simulink model "ANS_GFM_long_term"  (R2021b)
settings: Solver=FixedStepAuto  StartTime=0.0  StopTime=160  FixedStep=Ts  MaxStep=1e-5  RelTol=1e-3
values from neighbouring files (symbols this model uses):
  angle_load = angle(LF.bus(ind_l).Vbus)*180/pi    [init_ANS_GFM_long_term.m]    (also in init_ANS_GFM_short_term.m)
  angleV_LF = Vangle_init/180*pi    [init_ANS_GFM_long_term.m]    (also in init_ANS_GFM_short_term.m)
  awu = 1    [init_ANS_GFM_long_term.m]    (also in init_ANS_GFM_short_term.m)
  C_dc = 1/(Xcdc_pu_or*Zbase_dc_new*100*pi)    [init_ANS_GFM_long_term.m]    (also in init_ANS_GFM_short_term.m)
  C_f = 1/(Xcf_pu_or*Zbase_new*100*pi)    (= 0.013712)    [init_ANS_GFM_long_term.m]    (also in init_ANS_GFM_short_term.m = 0.0141333333333)
  control = 3    [init_ANS_GFM_long_term.m]    (also in init_ANS_GFM_short_term.m = 1)
  D_p = (1/(m_p*w_b))    (= 5209935.26289)    [init_ANS_GFM_long_term.m]    (also in init_ANS_GFM_short_term.m = 5370022.73304)
  Egrid_tmp = 1.054080675694902*400e3    (= 421632.270278)    [init_ANS_GFM_long_term.m]    (also in init_ANS_GFM_short_term.m)
  epsi = 1e-4    (= 0.0001)    [init_ANS_GFM_long_term.m]    (also in init_ANS_GFM_short_term.m)
  eta = m_p*V_m^2    [init_ANS_GFM_long_term.m]    (also in init_ANS_GFM_short_term.m)
  gamma = 2.3    [init_ANS_GFM_long_term.m]    (also in init_ANS_GFM_short_term.m)
  I0_init = [I0_init_a, I0_init_b, I0_init_c]    [init_ANS_GFM_long_term.m]    (also in init_ANS_GFM_short_term.m)
  I_bc = S_bc / (V_bc*sqrt(3))    [init_ANS_GFM_long_term.m]    (also in init_ANS_GFM_short_term.m)
  I_d_int_init = (U_d_int + I_q_int*L_f*w_b - V_d_int - I_d_int*R_f*0)    [init_ANS_GFM_long_term.m]    (also in init_ANS_GFM_short_term.m)
  I_init = [I_init_a, I_init_b, I_init_c]    [init_ANS_GFM_long_term.m]    (also in init_ANS_GFM_short_term.m)
  i_ll = -1.15*(S_bc/Vdc_n)-i_loss_dc    [init_ANS_GFM_long_term.m]    (also in init_ANS_GFM_short_term.m)
  I_max_sat_pu = 1.0 * I_bc *sqrt(2)    [init_ANS_GFM_long_term.m]    (also in init_ANS_GFM_short_term.m)
  I_q_int_init = (U_q_int - I_d_int*L_f*w_b - V_q_int - I_q_int*R_f*0)    [init_ANS_GFM_long_term.m]    (also in init_ANS_GFM_short_term.m)
  i_ul = 1.15*(S_bc/Vdc_n)+i_loss_dc    [init_ANS_GFM_long_term.m]    (also in init_ANS_GFM_short_term.m)
  idppu = 0.95    [init_ANS_GFM_long_term.m]    (also in init_ANS_GFM_short_term.m = 0.92)
  init_dP = -inv(A_pm)*B_pm*dP    [init_ANS_GFM_long_term.m]    (also in init_ANS_GFM_short_term.m)
  init_pm = -inv(A_pm)*B_pm*P_aft    [init_ANS_GFM_long_term.m]    (also in init_ANS_GFM_short_term.m)
  init_tau = -inv(A_tau)*B_tau*idc    [init_ANS_GFM_long_term.m]    (also in init_ANS_GFM_short_term.m)
  init_v1 = 1.0    (= 1)    [init_ANS_GFM_long_term.m]    (also in init_ANS_GFM_short_term.m)
  init_v2 = abs(LF.bus(ind_g).Vbus)/sqrt(2)    [init_ANS_GFM_long_term.m]    (also in init_ANS_GFM_short_term.m)
  init_v3 = abs(LF.bus(ind_sg).Vbus)/sqrt(2)    [init_ANS_GFM_long_term.m]    (also in init_ANS_GFM_short_term.m)
  init_vload = 1.0    (= 1)    [init_ANS_GFM_long_term.m]    (also in init_ANS_GFM_short_term.m)
  J = D_p*tau_f    (= 104198.705258)    [init_ANS_GFM_long_term.m]    (also in init_ANS_GFM_short_term.m = 107400.454661)
  k_dc = eta_1/(Vdc_n*m_p)    [init_ANS_GFM_long_term.m]    (also in init_ANS_GFM_short_term.m)
  K_p = (1/Vdc_n)    [init_ANS_GFM_long_term.m]    (also in init_ANS_GFM_short_term.m)
  K_r = 1/R_dc    [init_ANS_GFM_long_term.m]    (also in init_ANS_GFM_short_term.m)
  Kff_i = 1    [init_ANS_GFM_long_term.m]    (also in init_ANS_GFM_short_term.m)
  Kff_v = 1    [init_ANS_GFM_long_term.m]    (also in init_ANS_GFM_short_term.m)
  Ki_i = (1/n)*1.19    (= 0.0520711785298)    [init_ANS_GFM_long_term.m]    (also in init_ANS_GFM_short_term.m = 0.0505188679245)
  Ki_pll = 4255.3    [init_ANS_GFM_long_term.m]    (also in init_ANS_GFM_short_term.m)
  Ki_v = (n)*1.161022    (= 26.5332227733)    [init_ANS_GFM_long_term.m]    (also in init_ANS_GFM_short_term.m = 27.3485182222)
  ki_v_ac = 2*0.25    (= 0.5)    [init_ANS_GFM_long_term.m]    (also in init_ANS_GFM_short_term.m)
  Kp_i = 0.738891/n    (= 0.032331869895)    [init_ANS_GFM_long_term.m]    (also in init_ANS_GFM_short_term.m = 0.0313680141509)
  Kp_pll = 92    [init_ANS_GFM_long_term.m]    (also in init_ANS_GFM_short_term.m)
  Kp_v = 0.52*n    (= 11.8837333333)    [init_ANS_GFM_long_term.m]    (also in init_ANS_GFM_short_term.m = 12.2488888889)
  kp_v_ac = 0.001    [init_ANS_GFM_long_term.m]    (also in init_ANS_GFM_short_term.m)
  Kpl = 5.0    (= 5)    [init_ANS_GFM_long_term.m]    (also in init_ANS_GFM_short_term.m)
  L1 = cf/sqrt(1+RX^2)*(400e3)^2/Skss/(100*pi)    [init_ANS_GFM_long_term.m]    (also in init_ANS_GFM_short_term.m)
  L_f = Xlf_pu_or*Zbase_new/100/pi    (= 4.37572928821e-06)    [init_ANS_GFM_long_term.m]    (also in init_ANS_GFM_short_term.m = 4.24528301887e-06)
  Lf = 1e6/100/pi    (= 3183.09886184)    [init_ANS_GFM_long_term.m]    (also in init_ANS_GFM_short_term.m = 0.0636619772368)
  m_p = (2*pi*0.5)/(S_bc)    (= 6.10967066042e-10)    [init_ANS_GFM_long_term.m]    (also in init_ANS_GFM_short_term.m = 5.92753330866e-10)
  n = 1/Zb    (= 22.8533333333)    [init_ANS_GFM_long_term.m]    (also in init_ANS_GFM_short_term.m = 23.5555555556)
  P_LF_si = P_LF*S_b    [init_ANS_GFM_long_term.m]    (also in init_ANS_GFM_short_term.m)
  ps = 4440e6/S_bc    (= 0.863477246208)    [init_ANS_GFM_long_term.m]    (also in init_ANS_GFM_short_term.m = 0.837735849057)
  Q_LF_si = Q_LF*S_b    [init_ANS_GFM_long_term.m]    (also in init_ANS_GFM_short_term.m)
  qs = Q_LF*S_b/S_bc    [init_ANS_GFM_long_term.m]    (also in init_ANS_GFM_short_term.m)
  R1 = RX*cf/sqrt(1+RX^2)*(400e3)^2/Skss    [init_ANS_GFM_long_term.m]    (also in init_ANS_GFM_short_term.m)
  R_dc = Rdc_pu_or*Zbase_dc_new    [init_ANS_GFM_long_term.m]    (also in init_ANS_GFM_short_term.m)
  R_f = Rf_pu_or*Zbase_new    (= 2.18786464411e-05)    [init_ANS_GFM_long_term.m]    (also in init_ANS_GFM_short_term.m = 2.12264150943e-05)
  Rf = 1e6    (= 1000000)    [init_ANS_GFM_long_term.m]    (also in init_ANS_GFM_short_term.m = 20)
  S_bc = 5142e6    (= 5142000000)    [init_ANS_GFM_long_term.m]    (also in init_ANS_GFM_short_term.m = 5300000000)
  sat_select = 3    [init_ANS_GFM_long_term.m]    (also in init_ANS_GFM_short_term.m)
  SECM = 3    [init_ANS_GFM_long_term.m]    (also in init_ANS_GFM_short_term.m = 1)
  share_i_load = 1.0    (= 1)    [init_ANS_GFM_long_term.m]    (also in init_ANS_GFM_short_term.m)
  T_en = -0.5    [init_ANS_GFM_long_term.m]    (also in init_ANS_GFM_short_term.m)
  T_off = T_on + 0.1    (= 0.2)    [init_ANS_GFM_long_term.m]    (also in init_ANS_GFM_short_term.m)
  T_on = 0.1    [init_ANS_GFM_long_term.m]    (also in init_ANS_GFM_short_term.m)
  Ts = 2e-6    (= 2e-06)    [init_ANS_GFM_long_term.m]    (also in init_ANS_GFM_short_term.m = 1e-06)
  U_init = [Umag_init_a, Umag_init_b, Umag_init_c]    [init_ANS_GFM_long_term.m]    (also in init_ANS_GFM_short_term.m)
  Uangle_init = angle(V_LF_VSC)*180/pi    [init_ANS_GFM_long_term.m]    (also in init_ANS_GFM_short_term.m)
  Umag_init = abs(V_LF_VSC)*V_bc*sqrt(2/3)    [init_ANS_GFM_long_term.m]    (also in init_ANS_GFM_short_term.m)
  V1_rms = 15e3    (= 15000)    [init_ANS_GFM_long_term.m]    (also in init_ANS_GFM_short_term.m)
  V_d_int = abs(V_LF)*V_bc*sqrt(2/3)    [init_ANS_GFM_long_term.m]    (also in init_ANS_GFM_short_term.m)
  V_d_int_init = (I_d_int + V_q_int*C_f*w_b - I0_d_int)    [init_ANS_GFM_long_term.m]    (also in init_ANS_GFM_short_term.m)
  V_init = [V_init_a, V_init_b, V_init_c]    [init_ANS_GFM_long_term.m]    (also in init_ANS_GFM_short_term.m)
  V_m = sqrt(2/3)*V_bc    [init_ANS_GFM_long_term.m]    (also in init_ANS_GFM_short_term.m)
  V_q_int_init = (I_q_int - V_d_int*C_f*w_b - I0_q_int)    [init_ANS_GFM_long_term.m]    (also in init_ANS_GFM_short_term.m)
  Vdc_n = 3*V_m    [init_ANS_GFM_long_term.m]    (also in init_ANS_GFM_short_term.m)
  Vref = V_LF_mag*V_m    [init_ANS_GFM_long_term.m]    (also in init_ANS_GFM_short_term.m)
  w_b = 2*pi*f_b    (= 314.159265359)    [init_ANS_GFM_long_term.m]    (also in init_ANS_GFM_short_term.m)
  w_f = 2*pi*5    (= 31.4159265359)    [init_ANS_GFM_long_term.m]    (also in init_ANS_GFM_short_term.m)
  Zbase_new = V1_rms^2/S_bc    (= 0.0437572928821)    [init_ANS_GFM_long_term.m]    (also in init_ANS_GFM_short_term.m = 0.0424528301887)
undefined symbols (not defined in the file or in its folder): A_pm, A_tau, B_pm, B_tau, C_pm, C_tau, D_pm, D_tau, find_system, idq0_init, Pm, sm_init, v_d, v_q, Ve
libraries: spsBreakerLib x135, spsGroundLib x18, spsThreePhaseSeriesRLCBranchLib x12, spsabctodq0Lib x11, simulink x9, spsThreePhaseVIMeasurementLib x7, spsLoadFlowBusLib x7, spsSeriesRLCBranchLib x6, spsControlledVoltageSourceLib x6, spsCurrentMeasurementLib x6, spsVoltageMeasurementLib x6, spsRMSLib x5
(part 2 of 5)

== system ANS_GFM_long_term/OLTC ==
  note: G. Sybille, P. Giroux Hydro-Quebec (IREQ)
  note: This Three-Phase OLTC Regulating Transformer is built with three Multi-Winding Transformer blocks
      | and three On-Load Tap Changers (OLTC) subsystems using switches.
      | It implements a fixed number of taps (8 taps per phase +  tap 0 (nominal voltage ratio)).
      |
      | In order to change the number of taps you must modify the 3 Transformer blocks
      | and the 3  OLTC blocks as explained in the  the procedure given below:
  Vm (pu) : Inport
  " OLTC Control" : Subsystem  mask{NumberOfTaps=NumberOfTaps, TapSelectionTime=TapSelectionTime, TransferTime=TransferTime, InitialTap=InitialTap}
      mask prompts: NumberOfTaps "Number of taps:"; TapSelectionTime "Operating time of the tap selector (typical 3-10 s):"; TransferTime "Operating time of the transfer switch (typical 40-60 ms):"; InitialTap "Initial tap:"
      mask init:
      | TapVector=0:NumberOfTaps;
      | InitialStates=zeros(1,NumberOfTaps+1);
  Constant : Constant  Value=RegulatorOn
  Display : Display  Commented=on
  Goto Tag Visibility : GotoTagVisibility  GotoTag=SwSelect
  Goto Tag Visibility1 : GotoTagVisibility  GotoTag=SwTransfer
  Goto Tag Visibility2 : GotoTagVisibility  GotoTag=SwInversion
  Ground : spsGroundLib/Ground  LConnTagsString=a
  Ground1 : spsGroundLib/Ground  LConnTagsString=a
  Ground2 : spsGroundLib/Ground  LConnTagsString=a
  OLTCA : Subsystem  mask{NumberOfTaps=NumberOfTaps, InitialTap=InitialTap, Rtransfer=Rtransfer}
      mask prompts: NumberOfTaps "Nombre de prises:"; InitialTap "Prise initiale:"; Rtransfer "Resistance de court circuit (ohms):"
      mask init:
      | TapVector=0:NumberOfTaps;
      | InitialStates=zeros(1,NumberOfTaps+1);
      | InitialStates(abs(InitialTap)+1)=1;
      | 
      | InitialStateInv1=(InitialTap>=0);
      | InitialStateInv2=(InitialTap<0);
      | InitialStateInv3=InitialStateInv1;
      | InitialStateInv4=InitialStateInv2;
  OLTCA1 : Subsystem  mask{NumberOfTaps=NumberOfTaps, InitialTap=InitialTap, Rtransfer=Rtransfer}
      mask prompts: NumberOfTaps "Nombre de prises:"; InitialTap "Prise initiale:"; Rtransfer "Resistance de court circuit (ohms):"
      mask init: same as ANS_GFM_long_term/OLTC/OLTCA
  OLTCA2 : Subsystem  mask{NumberOfTaps=NumberOfTaps, InitialTap=InitialTap, Rtransfer=Rtransfer}
      mask prompts: NumberOfTaps "Nombre de prises:"; InitialTap "Prise initiale:"; Rtransfer "Resistance de court circuit (ohms):"
      mask init: same as ANS_GFM_long_term/OLTC/OLTCA
  OLTCA3 : Subsystem  Commented=on  mask{NumberOfTaps=NumberOfTaps, InitialTap=InitialTap, Rtransfer=Rtransfer}
      mask prompts: NumberOfTaps "Nombre de prises:"; InitialTap "Prise initiale:"; Rtransfer "Resistance de court circuit (ohms):"
      mask init: same as ANS_GFM_long_term/OLTC/OLTCA
  OLTCC1 : Subsystem  Commented=on  mask{NumberOfTaps=NumberOfTaps, InitialTap=InitialTap, Rtransfer=Rtransfer}
      mask prompts: NumberOfTaps "Nombre de prises:"; InitialTap "Prise initiale:"; Rtransfer "Resistance de court circuit (ohms):"
      mask init: same as ANS_GFM_long_term/OLTC/OLTCA
  Subsystem : Subsystem
      mask Display: disp('Procedure\n to change\n the number of taps')
  TransformerA : spsMultiWindingTransformerLib/Multi-Winding Transformer  LeftWindings=1  RightWindings=2  TappedWindings=taps on upper right winding  NumberOfTaps=19  SetSaturation=off  Hysteresis=off  DataFile='hysteresis.mat'  Measurements=None  UNITS=pu  NominalPower="[Pnom  Fnom]"  NominalVoltages=[Vnom1 VnomTaps Vnom2 ]  WindingResistances=[Rpu1 RpuTaps Rpu2]  WindingInductances="[Xpu1 XpuTaps  Xpu2 ]"  Rm=Rm  Lm=Lm  Saturation=[ 0,0 ; 0.0024,1.2 ; 1.0,1.52 ]  BreakLoop=off  DiscreteSolver=Trapezoidal iterative  DataType=off  InitialFlux=0  TransfoNumber=1
      settings: SourceProductBaseCode=PS
  TransformerB : spsMultiWindingTransformerLib/Multi-Winding Transformer  LeftWindings=1  RightWindings=2  TappedWindings=taps on upper right winding  NumberOfTaps=19  SetSaturation=off  Hysteresis=off  DataFile='hysteresis.mat'  Measurements=None  UNITS=pu  NominalPower="[Pnom  Fnom]"  NominalVoltages=[Vnom1 VnomTaps Vnom2 ]  WindingResistances=[Rpu1 RpuTaps Rpu2]  WindingInductances="[Xpu1 XpuTaps  Xpu2 ]"  Rm=Rm  Lm=Lm  Saturation=[ 0,0 ; 0.0024,1.2 ; 1.0,1.52 ]  BreakLoop=off  DiscreteSolver=Trapezoidal iterative  DataType=off  InitialFlux=0  TransfoNumber=1
      settings: SourceProductBaseCode=PS
  TransformerC : spsMultiWindingTransformerLib/Multi-Winding Transformer  LeftWindings=1  RightWindings=2  TappedWindings=taps on upper right winding  NumberOfTaps=19  SetSaturation=off  Hysteresis=off  DataFile='hysteresis.mat'  Measurements=None  UNITS=pu  NominalPower="[Pnom  Fnom]"  NominalVoltages=[Vnom1 VnomTaps Vnom2 ]  WindingResistances=[Rpu1 RpuTaps Rpu2]  WindingInductances="[Xpu1 XpuTaps  Xpu2 ]"  Rm=Rm  Lm=Lm  Saturation=[ 0,0 ; 0.0024,1.2 ; 1.0,1.52 ]  BreakLoop=off  DiscreteSolver=Trapezoidal iterative  DataType=off  InitialFlux=0  TransfoNumber=1
      settings: SourceProductBaseCode=PS
  Voltage regulator : Subsystem  mask{Vref=RegulatorVref, DeadBand=RegulatorDeadBand, TimeDelay=RegulatorDelay}
      mask prompts: Vref "Vref (pu)"; DeadBand "Deadband (pu)"; TimeDelay "Time delay (s)"
  A : PMIOPort  Tag=PMCPort  Side=Left
  B : PMIOPort  Tag=PMCPort  Port=2  Side=Left
  C : PMIOPort  Tag=PMCPort  Port=3  Side=Left
  a : PMIOPort  Tag=PMCPort  Port=4  Side=Right
  b : PMIOPort  Tag=PMCPort  Port=5  Side=Right
  c : PMIOPort  Tag=PMCPort  Port=6  Side=Right
  Tap : Outport  VectorParamsAs1DForOutWhenUnconnected=off
  tag scope: SwInversion=scoped, SwSelect=scoped, SwTransfer=scoped
  wires:
  Constant/1 -> Voltage regulator/3(RegOn)
  Vm (pu)/1 -> Voltage regulator/1(Vmes (pu))
  Voltage regulator/2(Down) -> " OLTC Control"/2(Down)
  " OLTC Control"/5(Ready) -> Voltage regulator/2(Ready)
  Voltage regulator/1(Up) -> " OLTC Control"/1(Up)
  " OLTC Control"/4(SwInv) -> [SwInversion]
  " OLTC Control"/1(Tap) -> Display/1, Tap/1  "Tap"
  " OLTC Control"/2(SwSelect) -> [SwSelect]
  " OLTC Control"/3(SwTr) -> [SwTransfer]
  connections:
  OLTCA/RConn22 -- TransformerA/RConn22
  OLTCA/RConn21 -- TransformerA/RConn21
  OLTCA/RConn20 -- TransformerA/RConn20
  OLTCA/RConn19 -- TransformerA/RConn19
  OLTCA/RConn18 -- TransformerA/RConn18
  OLTCA/RConn17 -- TransformerA/RConn17
  OLTCA/RConn16 -- TransformerA/RConn16
  OLTCA/RConn15 -- TransformerA/RConn15
  OLTCA/RConn13 -- TransformerA/RConn13
  OLTCA/RConn12 -- TransformerA/RConn12
  OLTCA/RConn14 -- TransformerA/RConn14
  OLTCA/RConn11 -- TransformerA/RConn11
  OLTCA/RConn10 -- TransformerA/RConn10
  OLTCA/RConn9 -- TransformerA/RConn9
  OLTCA/RConn8 -- TransformerA/RConn8
  OLTCA/RConn7 -- TransformerA/RConn7
  OLTCA/RConn6 -- TransformerA/RConn6
  OLTCA/RConn5 -- TransformerA/RConn5
  OLTCA/RConn4 -- TransformerA/RConn4
  OLTCA/RConn3 -- TransformerA/RConn3
  OLTCA/RConn2 -- TransformerA/RConn2
  OLTCA/RConn1 -- TransformerA/RConn1
  Ground/LConn1 -- TransformerA/RConn23
  OLTCA/LConn1 -- a/RConn1
  Ground1/LConn1 -- TransformerB/RConn23
  OLTCA1/RConn7 -- TransformerB/RConn7
  OLTCA1/RConn17 -- TransformerB/RConn17
  OLTCA1/RConn21 -- TransformerB/RConn21
  OLTCA1/RConn15 -- TransformerB/RConn15
  OLTCA1/RConn14 -- TransformerB/RConn14
  OLTCA1/RConn3 -- TransformerB/RConn3
  OLTCA1/RConn9 -- TransformerB/RConn9
  OLTCA1/RConn13 -- TransformerB/RConn13
  OLTCA1/RConn8 -- TransformerB/RConn8
  OLTCA1/RConn1 -- TransformerB/RConn1
  OLTCA1/RConn16 -- TransformerB/RConn16
  OLTCA1/RConn12 -- TransformerB/RConn12
  OLTCA1/RConn4 -- TransformerB/RConn4
  OLTCA1/RConn5 -- TransformerB/RConn5
  OLTCA1/RConn2 -- TransformerB/RConn2
  OLTCA1/RConn10 -- TransformerB/RConn10
  OLTCA1/RConn6 -- TransformerB/RConn6
  OLTCA1/RConn20 -- TransformerB/RConn20
  OLTCA1/RConn22 -- TransformerB/RConn22
  OLTCA1/RConn18 -- TransformerB/RConn18
  OLTCA1/RConn19 -- TransformerB/RConn19
  OLTCA1/RConn11 -- TransformerB/RConn11
  Ground2/LConn1 -- TransformerC/RConn23
  OLTCA2/RConn7 -- TransformerC/RConn7
  OLTCA2/RConn17 -- TransformerC/RConn17
  OLTCA2/RConn21 -- TransformerC/RConn21
  OLTCA2/RConn15 -- TransformerC/RConn15
  OLTCA2/RConn14 -- TransformerC/RConn14
  OLTCA2/RConn3 -- TransformerC/RConn3
  OLTCA2/RConn9 -- TransformerC/RConn9
  OLTCA2/RConn13 -- TransformerC/RConn13
  OLTCA2/RConn8 -- TransformerC/RConn8
  OLTCA2/RConn1 -- TransformerC/RConn1
  OLTCA2/RConn16 -- TransformerC/RConn16
  OLTCA2/RConn12 -- TransformerC/RConn12
  OLTCA2/RConn4 -- TransformerC/RConn4
  OLTCA2/RConn5 -- TransformerC/RConn5
  OLTCA2/RConn2 -- TransformerC/RConn2
  OLTCA2/RConn10 -- TransformerC/RConn10
  OLTCA2/RConn6 -- TransformerC/RConn6
  OLTCA2/RConn20 -- TransformerC/RConn20
  OLTCA2/RConn22 -- TransformerC/RConn22
  OLTCA2/RConn18 -- TransformerC/RConn18
  OLTCA2/RConn19 -- TransformerC/RConn19
  OLTCA2/RConn11 -- TransformerC/RConn11
  OLTCA2/LConn1 -- c/RConn1
  OLTCA1/LConn1 -- b/RConn1
  TransformerA/LConn2 -- TransformerB/LConn1 -- B/RConn1
  TransformerB/LConn2 -- C/RConn1 -- TransformerC/LConn1
  TransformerC/LConn2 -- A/RConn1 -- TransformerA/LConn1

== system ANS_GFM_long_term/Synchronous Generator(GENTPJ) ==
  ve : Inport
  Pm : Inport  Port=2
  AVR+OEL+PSS : Subsystem  mask(AVR){ve0=Ve, uref=1.0, ifdlim=3.0618, L1=-20, L2=5, G=120, Ta=5, Tb=12.5, PSS_act=1, Kp=75, Tw=15, T1=0.22, T2=0.012, C=0.1}
      mask prompts: ve0 "Initialisierung Erregerspannung (ve0)"; uref "Referenzklemmenspannung (uref)"; ifdlim "max. Erregerstrom (ifdlim)"; L1 "Over-Excitation Limit (L1)"; L2 "AVR Limit (L2)"; G "Verstärkungsfaktor (G)"; Ta "AVR Zeitkonstante (Ta)"; Tb "AVR Zeitkonstante (Tb)"; PSS_act "PSS on/off (1/0)"; Kp "Verstärkungsfaktor PSS"; Tw "Wash-Out Filter (Tw)"; T1 "PSS Zeitkonstante (T1)"; T2 "PSS Zeitkonstante (T2)"; C "PSS Begrenzung"
      mask help: AVR
  Grid Interface : Subsystem
  Mechanical Equations : Subsystem
  Power calculation : Subsystem
  Rotor Equations : Subsystem
  Stator Equations : Subsystem
  Terminator : Terminator
  To Workspace1 : ToWorkspace  VariableName=psm  SampleTime=-1
      settings: Decimation=100
  To Workspace2 : ToWorkspace  VariableName=ifdsm  SampleTime=-1
      settings: Decimation=100
  a : PMIOPort  Side=Right
  b : PMIOPort  Port=2  Side=Right
  c : PMIOPort  Port=3  Side=Right
  delta : Outport
  wt : Outport  Port=2
  wires:
  Mechanical Equations/1(1+w) -> AVR+OEL+PSS/3(xspeed), Stator Equations/6(1+w), Power calculation/1(1+w)
  Stator Equations/2(Vqterm) -> Grid Interface/2(Vqterm), Power calculation/3(Vqterm)
  Power calculation/1(Te) -> To Workspace1/1, Mechanical Equations/2(Te)
  Rotor Equations/1(ifd) -> AVR+OEL+PSS/1(ie), To Workspace2/1
  Mechanical Equations/2(wt) -> Grid Interface/3(wt), wt/1
  Mechanical Equations/3(delta) -> delta/1
  Pm/1 -> Mechanical Equations/1(Pm)
  Rotor Equations/2(Edss) -> Stator Equations/3(Edss)
  Rotor Equations/3(Eqss) -> Stator Equations/4(Eqss)
  Grid Interface/1(id) -> Power calculation/4(Id), Stator Equations/1(Id), Rotor Equations/2(id)
  Grid Interface/2(iq) -> Power calculation/5(Iq), Stator Equations/2(Iq), Rotor Equations/3(iq)
  Grid Interface/4(|Uterm|) -> AVR+OEL+PSS/2(ut)
  ve/1 -> Terminator/1
  Stator Equations/1(Vdterm) -> Grid Interface/1(Vdterm), Power calculation/2(Vdterm)  "Eqs"
  Grid Interface/3(El) -> Stator Equations/5(E_l), Rotor Equations/4(El)
  AVR+OEL+PSS/1(ve) -> Rotor Equations/1(ve)
  connections:
  Grid Interface/RConn1 -- a/RConn1
  Grid Interface/RConn3 -- c/RConn1
  Grid Interface/RConn2 -- b/RConn1

== system ANS_GFM_long_term/Constant Current Load (EMT)/PLL ==
  Vabc : Inport
  Constant1 : Constant  Value=sqrt(2)*Pload/(sqrt(3)*Urms)
  Constant2 : Constant  Value=0
  Constant4 : Constant  Value=100*pi
  Cos : Trigonometry  Operator=cos
  Cos1 : Trigonometry
  Demux1 : Demux  Outputs=3
  Demux2 : Demux  Outputs=3
  Gain4 : Gain  Gain=Ki
  Gain5 : Gain  Gain=Kp
  Integrator2 : Integrator  InitialCondition=angle_load/180*pi-pi/2
  Integrator3 : Integrator
  Mux : Mux  Inputs=3
  Product : Product
  Product1 : Product
  Saturation1 : Saturate  UpperLimit=2*pi*55  LowerLimit=2*pi*45
  Sum2 : Sum  Inputs=|++
  Sum3 : Sum  Inputs=|++
  Sum4 : Sum  Inputs=-+
  Terminator : Terminator
  abc to Alpha-Beta-Zero : spsabctoAlphaBetaZeroLib/abc to Alpha-Beta-Zero
      settings: SourceProductBaseCode=PS
  delay : TransferFcn  Denominator=[Ts 1]
  dq0 to abc : spsdq0toabcLib/dq0 to abc  Alignment=Aligned with phase A axis
  Ia : Outport
  Ib : Outport  Port=2
  Ic : Outport  Port=3
  wires:
  Demux1/1 -> Ia/1
  Demux1/2 -> Ib/1
  Mux/1 -> dq0 to abc/1
  dq0 to abc/1 -> Demux1/1
  Demux1/3 -> Ic/1
  Constant2/1 -> Mux/2, Mux/3
  Constant1/1 -> Mux/1
  abc to Alpha-Beta-Zero/1 -> Demux2/1
  Sum2/1 -> Sum3/1
  Integrator3/1 -> Sum2/2
  Saturation1/1 -> Integrator2/1
  Gain5/1 -> Sum2/1
  Sum3/1 -> Saturation1/1
  Gain4/1 -> Integrator3/1
  Constant4/1 -> Sum3/2
  Product/1 -> Sum4/1
  Product1/1 -> Sum4/2
  Integrator2/1 -> Cos1/1, Cos/1, dq0 to abc/2
  Cos/1 -> Product1/2
  Cos1/1 -> Product/1
  Vabc/1 -> abc to Alpha-Beta-Zero/1
  Demux2/1 -> Product/2
  Demux2/2 -> Product1/1
  Sum4/1 -> delay/1
  delay/1 -> Gain4/1, Gain5/1
  Demux2/3 -> Terminator/1

== system ANS_GFM_long_term/GFM Converter/Converter (modified by S. Liemann) ==
  note: AC sources
  Vdq0 : Inport
  Pe_ac : Inport  Port=2
  Idc : Inport  Port=3
  wt : Inport  Port=4
  Divide : Product  Inputs=*/
  Gain12 : Gain  Gain=1/C_dc
  Gain13 : Gain  Gain=1/R_dc
  Gain8 : Gain  Gain=1/Vdc_n
  Integrator1 : Integrator  InitialCondition=Vdc_n
  Product5 : Product
  Subsystem1 : Subsystem
  Sum3 : Sum  Inputs=-+-
  dq0 to abc1 : spsdq0toabcLib/dq0 to abc  Alignment=90 degrees behind phase A axis
  a : PMIOPort  Side=Right
  b : PMIOPort  Port=2  Side=Right
  c : PMIOPort  Port=3  Side=Right
  Udc : Outport
  wires:
  Integrator1/1 -> Gain8/1, Divide/2, Udc/1, Gain13/1  "Udc"
  wt/1 -> dq0 to abc1/2
  Product5/1 -> dq0 to abc1/1
  Sum3/1 -> Gain12/1  "Ic"
  dq0 to abc1/1 -> Subsystem1/1(Vabc)
  Idc/1 -> Sum3/2
  Gain12/1 -> Integrator1/1
  Gain13/1 -> Sum3/3
  Vdq0/1 -> Product5/1
  Pe_ac/1 -> Divide/1
  Divide/1 -> Sum3/1
  Gain8/1 -> Product5/2
  connections:
  Subsystem1/RConn2 -- b/RConn1
  Subsystem1/RConn1 -- a/RConn1
  Subsystem1/RConn3 -- c/RConn1

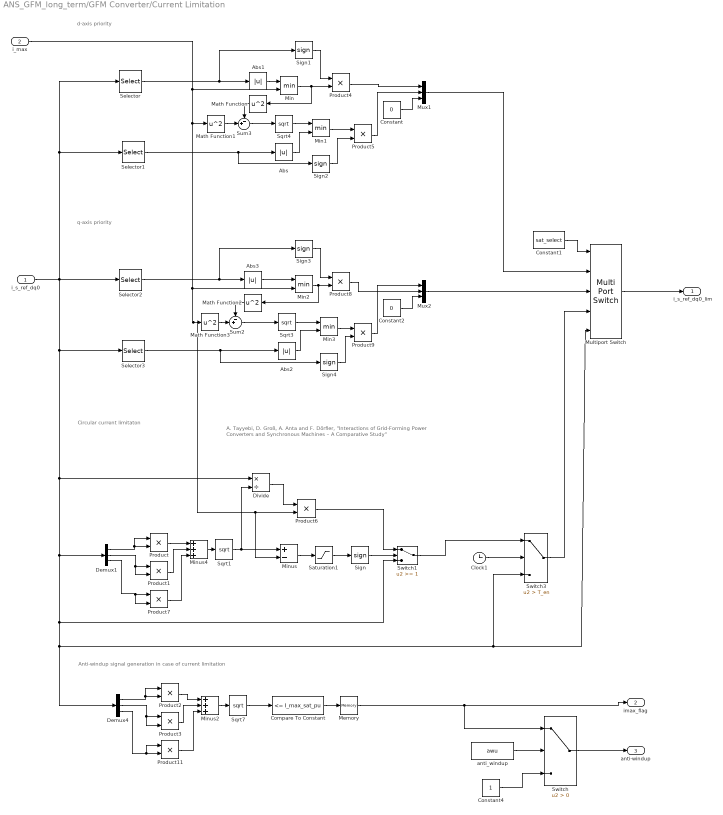
== system ANS_GFM_long_term/GFM Converter/Current Limitation ==
  note: Anti-windup signal generation in case of current limitation
  note: d-axis priority
  note: Circular current limitaton
  note: A. Tayyebi, D. Groß, A. Anta and F. Dörfler, "Interactions of Grid-Forming Power Converters and Synchronous Machines – A Comparative Study"
  note: q-axis priority
  i_s_ref_dq0 : Inport
  i_max : Inport  Port=2
  Abs{,1..3} (4 alike) : Abs
  Clock1 : Clock
  Compare To Constant : simulink/Logic and Bit Operations/Compare To Constant  relop=<=  const=I_max_sat_pu  OutDataTypeStr=boolean
  Constant : Constant  Value=0
  Constant1 : Constant  Value=sat_select
  Constant2 : Constant  Value=0
  Constant4 : Constant
  Demux1 : Demux  Outputs=3
  Demux4 : Demux  Outputs=3
  Divide : Product  Inputs=*/
  Math Function{,1..3} (4 alike) : Math  Operator=square  SaturateOnIntegerOverflow=on
  Memory : Memory  InitialCondition=1
  Min{,1..3} (4 alike) : MinMax  Inputs=2
  Minus : Sum  Inputs=+-
  Minus2 : Sum  Inputs=+++
  Minus4 : Sum  Inputs=+++
  Multiport Switch : MultiPortSwitch  Inputs=4
  Mux1 : Mux  Inputs=3
  Mux2 : Mux  Inputs=3
  Product{,1..3,6..7,11} (7 alike) : Product  RndMeth=Zero
  Product{4..5,8..9} (4 alike) : Product
  Saturation1 : Saturate  UpperLimit=inf  LowerLimit=0
  Selector : Selector  InputPortWidth=3  IndexOptions=Index vector (dialog)  Indices=[1 ]  OutputSizes=1
  Selector1 : Selector  InputPortWidth=3  IndexOptions=Index vector (dialog)  Indices=[2 ]  OutputSizes=1
  Selector2 : Selector  InputPortWidth=3  IndexOptions=Index vector (dialog)  Indices=[2 ]  OutputSizes=1
  Selector3 : Selector  InputPortWidth=3  IndexOptions=Index vector (dialog)  Indices=[1 ]  OutputSizes=1
  Sign{,1..4} (5 alike) : Signum
  Sqrt{1,3..4,7} (4 alike) : Sqrt  SaturateOnIntegerOverflow=on
  Sum2 : Sum  Inputs=-+|
  Sum3 : Sum  Inputs=-+|
  Switch : Switch  Criteria=u2 > Threshold
  Switch1 : Switch  Threshold=1
  Switch3 : Switch  Criteria=u2 > Threshold  Threshold=T_en
  anti_windup : Constant  Value=awu
  i_s_ref_dq0_lim : Outport  VectorParamsAs1DForOutWhenUnconnected=off
  imax_flag : Outport  Port=2
  anti-windup : Outport  Port=3
  wires:
  Demux1/3 -> Product7/2, Product7/1
  Product/1 -> Minus4/1
  Demux1/2 -> Product1/2, Product1/1
  Sqrt1/1 -> Minus/1, Divide/2
  Minus/1 -> Saturation1/1
  Demux1/1 -> Product/1, Product/2
  Product1/1 -> Minus4/2
  Minus4/1 -> Sqrt1/1
  Divide/1 -> Product6/1
  Saturation1/1 -> Sign/1
  Sign/1 -> Switch1/2
  Product7/1 -> Minus4/3
  Product6/1 -> Switch1/1
  Selector/1 -> Sign1/1, Abs1/1
  Sqrt4/1 -> Min1/1
  Sum3/1 -> Sqrt4/1
  Constant/1 -> Mux1/3
  Constant1/1 -> Multiport Switch/1
  Mux1/1 -> Multiport Switch/2
  Abs/1 -> Min1/2
  Selector1/1 -> Sign2/1, Abs/1
  Abs1/1 -> Min/1
  Sign1/1 -> Product4/1
  Min/1 -> Math Function/1, Product4/2
  Product4/1 -> Mux1/1
  Min1/1 -> Product5/1
  Product5/1 -> Mux1/2
  Sign2/1 -> Product5/2
  Sum2/1 -> Sqrt3/1
  Constant2/1 -> Mux2/3
  Product9/1 -> Mux2/1
  Selector3/1 -> Sign4/1, Abs2/1
  Abs2/1 -> Min3/2
  Sqrt3/1 -> Min3/1
  Selector2/1 -> Sign3/1, Abs3/1
  Abs3/1 -> Min2/1
  Product8/1 -> Mux2/2
  Sign4/1 -> Product9/2
  Min2/1 -> Math Function2/1, Product8/2
  Sign3/1 -> Product8/1
  Min3/1 -> Product9/1
  i_max/1 -> Math Function1/1, Minus/2, Product6/2, Math Function3/1, Min2/2, Min/2
  Mux2/1 -> Multiport Switch/3
  Math Function1/1 -> Sum3/2
  Math Function/1 -> Sum3/1
  Math Function3/1 -> Sum2/2
  Math Function2/1 -> Sum2/1
  Multiport Switch/1 -> i_s_ref_dq0_lim/1
  Minus2/1 -> Sqrt7/1
  Demux4/2 -> Product3/2, Product3/1
  Demux4/3 -> Product11/2, Product11/1
  Product3/1 -> Minus2/2
  Product11/1 -> Minus2/3
  Product2/1 -> Minus2/1
  Compare To Constant/1 -> Memory/1
  Demux4/1 -> Product2/1, Product2/2
  Sqrt7/1 -> Compare To Constant/1
  Switch/1 -> anti-windup/1
  Constant4/1 -> Switch/3
  anti_windup/1 -> Switch/2
  Switch1/1 -> Switch3/1
  Clock1/1 -> Switch3/2
  i_s_ref_dq0/1 -> Selector2/1, Selector1/1, Selector/1, Selector3/1, Switch3/3, Multiport Switch/5, Demux4/1, Switch1/3, Demux1/1, Divide/1
  Switch3/1 -> Multiport Switch/4
  Memory/1 -> imax_flag/1, Switch/1

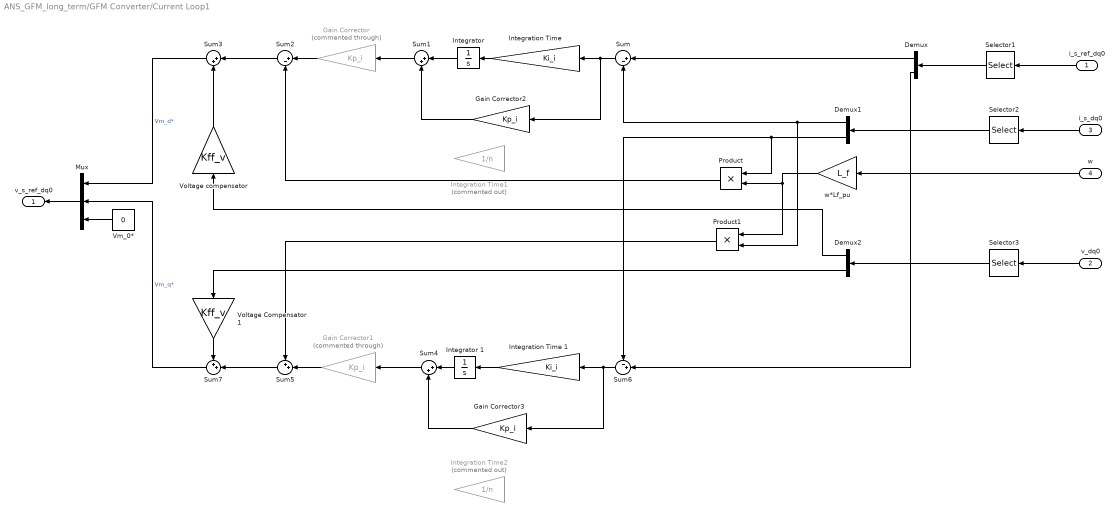
== system ANS_GFM_long_term/GFM Converter/Current Loop1 ==
  i_s_ref_dq0 : Inport
  v_dq0 : Inport  Port=2
  i_s_dq0 : Inport  Port=3
  w : Inport  Port=4
  Demux : Demux  Outputs=2
  Demux1 : Demux  Outputs=2
  Demux2 : Demux  Outputs=2
  Gain Corrector : Gain  Commented=through  Gain=Kp_i
  Gain Corrector1 : Gain  Commented=through  Gain=Kp_i
  Gain Corrector2 : Gain  Gain=Kp_i
  Gain Corrector3 : Gain  Gain=Kp_i
  Integration Time : Gain  Gain=Ki_i
  Integration Time 1 : Gain  Gain=Ki_i
  Integration Time1 : Gain  Commented=on  Gain=1/n
  Integration Time2 : Gain  Commented=on  Gain=1/n
  Integrator : Integrator  InitialCondition=I_d_int_init
  Integrator 1 : Integrator  InitialCondition=I_q_int_init
  Mux : Mux  Inputs=3
  Product : Product  RndMeth=Zero
  Product1 : Product  RndMeth=Zero
  Selector1 : Selector  InputPortWidth=3  IndexOptions=Index vector (dialog)  Indices=[1 2]  OutputSizes=1
  Selector2 : Selector  InputPortWidth=3  IndexOptions=Index vector (dialog)  Indices=[1 2]  OutputSizes=1
  Selector3 : Selector  InputPortWidth=3  IndexOptions=Index vector (dialog)  Indices=[1 2]  OutputSizes=1
  Sum : Sum  Inputs=|+-
  Sum1 : Sum  Inputs=|++
  Sum2 : Sum  Inputs=|+-
  Sum3 : Sum  Inputs=|++
  Sum4 : Sum  Inputs=|++
  Sum5 : Sum  Inputs=++|
  Sum6 : Sum  Inputs=-+|
  Sum7 : Sum  Inputs=++|
  Vm_0* : Constant  Value=0
  Voltage Compensator 1 : Gain  Gain=Kff_v
  Voltage compensator : Gain  Gain=Kff_v
  w*Lf_pu : Gain  Gain=L_f
  v_s_ref_dq0 : Outport  VectorParamsAs1DForOutWhenUnconnected=off
  wires:
  Gain Corrector1/1 -> Sum5/2
  Product1/1 -> Sum5/1
  Demux2/1 -> Voltage compensator/1
  Demux1/1 -> Sum/2, Product1/2
  Integrator/1 -> Sum1/1
  Vm_0*/1 -> Mux/3
  Demux1/2 -> Sum6/1, Product/1
  Selector3/1 -> Demux2/1
  i_s_dq0/1 -> Selector2/1
  Selector2/1 -> Demux1/1
  Mux/1 -> v_s_ref_dq0/1
  w/1 -> w*Lf_pu/1
  Gain Corrector/1 -> Sum2/1
  Selector1/1 -> Demux/1
  Demux/2 -> Sum6/2
  Sum4/1 -> Gain Corrector1/1
  Sum2/1 -> Sum3/1
  Sum1/1 -> Gain Corrector/1
  Voltage compensator/1 -> Sum3/2
  Integrator 1/1 -> Sum4/1
  v_dq0/1 -> Selector3/1
  i_s_ref_dq0/1 -> Selector1/1
  w*Lf_pu/1 -> Product/2, Product1/1
  Product/1 -> Sum2/2
  Voltage Compensator 1/1 -> Sum7/1
  Demux2/2 -> Voltage Compensator 1/1
  Sum7/1 -> Mux/2  "Vm_q*"
  Sum3/1 -> Mux/1  "Vm_d*"
  Demux/1 -> Sum/1
  Sum6/1 -> Integration Time 1/1, Gain Corrector3/1
  Sum5/1 -> Sum7/2
  Integration Time/1 -> Integrator/1
  Integration Time 1/1 -> Integrator 1/1
  Sum/1 -> Integration Time/1, Gain Corrector2/1
  Gain Corrector2/1 -> Sum1/2
  Gain Corrector3/1 -> Sum4/2

== system ANS_GFM_long_term/GFM Converter/GFM controls ==
  chosen_control : Inport
  P_abc : Inport  Port=2
  P_set : Inport  Port=3
  v_abc : Inport  Port=4
  v_dc : Inport  Port=5
  Q_abc : Inport  Port=6
  dv_q : Inport  Port=7
  Q_set : Inport  Port=8
  anti-windup : Inport  Port=9
  Compare To Constant1 : simulink/Logic and Bit Operations/Compare To Constant  relop===  const=1  OutDataTypeStr=boolean
  Compare To Constant2 : simulink/Logic and Bit Operations/Compare To Constant  relop===  const=2  OutDataTypeStr=boolean
  Compare To Constant3 : simulink/Logic and Bit Operations/Compare To Constant  relop===  const=3  OutDataTypeStr=boolean
  Compare To Constant4 : simulink/Logic and Bit Operations/Compare To Constant  relop===  const=4  OutDataTypeStr=boolean
  Constant : Constant  Value=w_b
  Constant1 : Constant  Value=Vref
  Demux : Demux  Outputs=3
  Droop Control : Subsystem
  Matching Control : Subsystem
  Multiport Switch : MultiPortSwitch  Inputs=4
  Mux{,1..3} (4 alike) : Mux  Inputs=3
  VSM Control : Subsystem
  dVOC  - kappa=pi/2 : Subsystem
  w_ref : Outport
  theta_ref : Outport  Port=2
  v_ref_dqo : Outport  Port=3
  wires:
  Droop Control/1(w_ref) -> Mux/1
  Droop Control/2(theta_ref) -> Mux/2
  Droop Control/3(v_ref_dq0) -> Mux/3
  Compare To Constant1/1 -> Droop Control/Enable
  Compare To Constant2/1 -> Matching Control/Enable
  Compare To Constant3/1 -> dVOC  - kappa=pi/2/Enable
  Compare To Constant4/1 -> VSM Control/Enable
  Constant/1 -> Droop Control/1(w_b), VSM Control/5(w_b), dVOC  - kappa=pi/2/1(w_b)
  Constant1/1 -> VSM Control/3(v_m), dVOC  - kappa=pi/2/4(v_m), Matching Control/3(v_m), Droop Control/4(v_m)
  Matching Control/1(w_ref) -> Mux1/1
  Matching Control/3(v_ref_dq0) -> Mux1/3
  Matching Control/2(theta_ref) -> Mux1/2
  dVOC  - kappa=pi/2/1(w_ref) -> Mux2/1
  dVOC  - kappa=pi/2/3(v_ref_dq0) -> Mux2/3
  dVOC  - kappa=pi/2/2(theta_ref) -> Mux2/2
  VSM Control/1(w_ref) -> Mux3/1
  VSM Control/3(v_ref_dq0) -> Mux3/3
  VSM Control/2(theta_ref) -> Mux3/2
  Multiport Switch/1 -> Demux/1
  Demux/1 -> w_ref/1
  Demux/2 -> theta_ref/1
  Demux/3 -> v_ref_dqo/1
  Mux3/1 -> Multiport Switch/5
  Mux2/1 -> Multiport Switch/4
  Mux1/1 -> Multiport Switch/3
  Mux/1 -> Multiport Switch/2
  P_abc/1 -> VSM Control/1(p_m), dVOC  - kappa=pi/2/2(p_m), Droop Control/2(p_m)
  v_abc/1 -> Matching Control/2(V_abc), Droop Control/5(V_abc), VSM Control/4(V_abc)
  v_dc/1 -> Matching Control/1(v_dc)
  Q_abc/1 -> dVOC  - kappa=pi/2/5(q_m)
  P_set/1 -> Droop Control/3(p_set), VSM Control/2(p_set), dVOC  - kappa=pi/2/3(p_set)
  anti-windup/1 -> Droop Control/6(anti-windup), Matching Control/4(anti-windup), dVOC  - kappa=pi/2/7(anti-windup), VSM Control/6(anti-windup)
  Q_set/1 -> dVOC  - kappa=pi/2/6(q_set)
  chosen_control/1 -> Compare To Constant4/1, Compare To Constant3/1, Compare To Constant2/1, Multiport Switch/1, Compare To Constant1/1
  dv_q/1 -> VSM Control/7(dv_q), dVOC  - kappa=pi/2/8(dv_q), Matching Control/5(dv_q), Droop Control/7(dv_q)

== system ANS_GFM_long_term/GFM Converter/PT1 ==
  in : Inport
  Gain15 : Gain  Gain=1/1e-4
  Integrator : Integrator  InitialCondition=ps*S_bc
  Sum6 : Sum  Inputs=|+-
  out : Outport
  wires:
  Integrator/1 -> out/1, Sum6/2
  Gain15/1 -> Integrator/1
  Sum6/1 -> Gain15/1
  in/1 -> Sum6/1

== system ANS_GFM_long_term/GFM Converter/PT2 ==
  in : Inport
  Gain15 : Gain  Gain=1/1e-4
  Integrator : Integrator
  Sum6 : Sum  Inputs=|+-
  out : Outport
  wires:
  Integrator/1 -> out/1, Sum6/2
  Gain15/1 -> Integrator/1
  Sum6/1 -> Gain15/1
  in/1 -> Sum6/1

== system ANS_GFM_long_term/GFM Converter/PT3 ==
  in : Inport
  Gain15 : Gain  Gain=1/1e-4
  Integrator : Integrator  InitialCondition=qs*S_bc
  Sum6 : Sum  Inputs=|+-
  out : Outport
  wires:
  Integrator/1 -> out/1, Sum6/2
  Gain15/1 -> Integrator/1
  Sum6/1 -> Gain15/1
  in/1 -> Sum6/1

== system ANS_GFM_long_term/GFM Converter/SECMs ==
  secm : Inport
  pset : Inport  Port=2
  imax_flag : Inport  Port=3
  V_dq0 : Inport  Port=4
  i_dqlim : Inport  Port=5
  i_s_dq0 : Inport  Port=6
  qset0 : Inport  Port=7
  Compare To Constant1 : simulink/Logic and Bit Operations/Compare To Constant  relop===  const=1  OutDataTypeStr=boolean
  Compare To Constant2 : simulink/Logic and Bit Operations/Compare To Constant  relop===  const=2  OutDataTypeStr=boolean
  Compare To Constant3 : simulink/Logic and Bit Operations/Compare To Constant  relop===  const=3  OutDataTypeStr=boolean
  Compare To Constant4 : simulink/Logic and Bit Operations/Compare To Constant  relop===  const=4  OutDataTypeStr=boolean
  Demux : Demux  Outputs=3
  Gain : Gain  Gain=1/V_m
  Gain1 : Gain  Gain=1/V_m
  Multiport Switch : MultiPortSwitch  Inputs=5
  Multiport Switch1 : MultiPortSwitch  Inputs=5
  SECM-1 : Subsystem
  SECM-2 : Subsystem
  SECM-3 : Subsystem
  SECM-4 : Subsystem
  Square : Math  Operator=square  SaturateOnIntegerOverflow=on
  Square Root : Sqrt  SaturateOnIntegerOverflow=on
  Sum of Elements : Sum  Inputs=+
  pset* : Outport
  dv_q : Outport  Port=2
  qset* : Outport  Port=3
  wires:
  secm/1 -> Compare To Constant3/1, Compare To Constant4/1, Compare To Constant2/1, Compare To Constant1/1, Multiport Switch1/1, Multiport Switch/1
  Multiport Switch/1 -> pset*/1
  Square/1 -> Sum of Elements/1
  Sum of Elements/1 -> Square Root/1
  Square Root/1 -> Gain/1
  Demux/2 -> Gain1/1
  SECM-3/2(dv_q) -> dv_q/1
  V_dq0/1 -> SECM-1/3(Vdq0), Square/1, Demux/1
  Multiport Switch1/1 -> qset*/1
  Compare To Constant1/1 -> SECM-1/Enable
  Compare To Constant2/1 -> SECM-2/Enable
  Compare To Constant3/1 -> SECM-3/Enable
  Compare To Constant4/1 -> SECM-4/Enable
  SECM-4/1(pset*) -> Multiport Switch/5
  SECM-3/1(pset*) -> Multiport Switch/4
  SECM-2/1(pset*) -> Multiport Switch/3
  SECM-1/1(pset*) -> Multiport Switch/2
  SECM-1/2(qset*) -> Multiport Switch1/2
  qset0/1 -> SECM-1/5(Qset0), Multiport Switch1/4, Multiport Switch1/5, Multiport Switch1/6, Multiport Switch1/3
  imax_flag/1 -> SECM-1/2(imax_flag)
  i_dqlim/1 -> SECM-1/4(Idq0_lim)
  pset/1 -> Multiport Switch/6, SECM-4/1(pset), SECM-3/1(pset), SECM-2/1(pset), SECM-1/1(Pset0)
  Gain1/1 -> SECM-3/2(V_q_pu)
  i_s_dq0/1 -> SECM-4/2(i_s_dq0)
  Gain/1 -> SECM-2/2(V_pu)

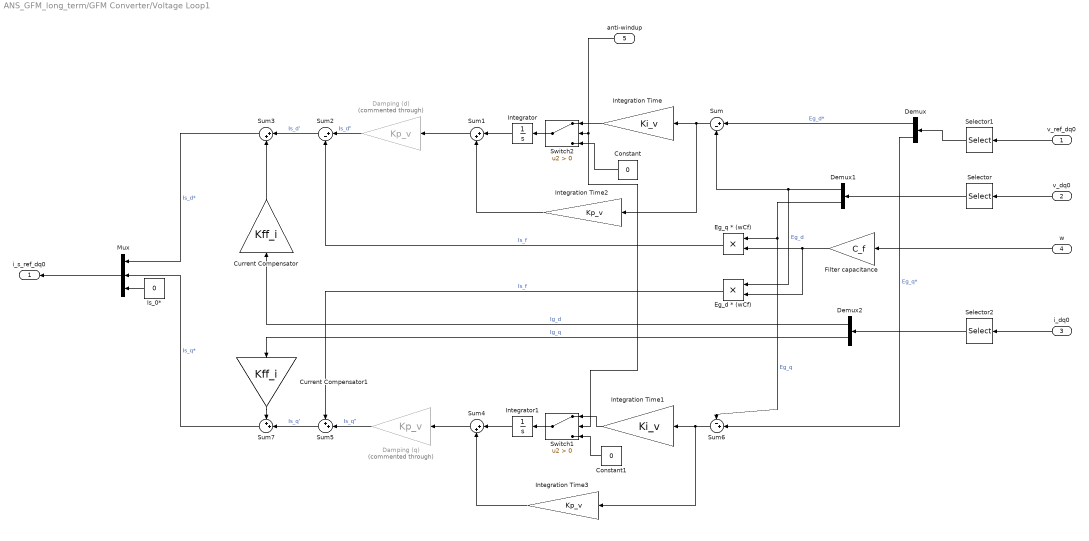
== system ANS_GFM_long_term/GFM Converter/Voltage Loop1 ==
  v_ref_dq0 : Inport
  v_dq0 : Inport  Port=2
  i_dq0 : Inport  Port=3
  w : Inport  Port=4
  anti-windup : Inport  Port=5
  Constant : Constant  Value=0
  Constant1 : Constant  Value=0
  Current Compensator : Gain  Gain=Kff_i
  Current Compensator1 : Gain  Gain=Kff_i
  Damping (d) : Gain  Commented=through  Gain=Kp_v
  Damping (q) : Gain  Commented=through  Gain=Kp_v
  Demux : Demux  Outputs=2
  Demux1 : Demux  Outputs=2
  Demux2 : Demux  Outputs=2
  Eg_d * (wCf) : Product  RndMeth=Zero
  "Eg_q * (wCf) " : Product  RndMeth=Zero
  Filter capacitance : Gain  Gain=C_f
  Integration Time : Gain  Gain=Ki_v
  Integration Time1 : Gain  Gain=Ki_v
  Integration Time2 : Gain  Gain=Kp_v
  Integration Time3 : Gain  Gain=Kp_v
  Integrator : Integrator  InitialCondition=V_d_int_init
  Integrator1 : Integrator  InitialCondition=V_q_int_init
  Is_0* : Constant  Value=0
  Mux : Mux  Inputs=3
  Selector : Selector  InputPortWidth=3  IndexOptions=Index vector (dialog)  Indices=[1 2]  OutputSizes=1
  Selector1 : Selector  InputPortWidth=3  IndexOptions=Index vector (dialog)  Indices=[1 2]  OutputSizes=1
  Selector2 : Selector  InputPortWidth=3  IndexOptions=Index vector (dialog)  Indices=[1 2]  OutputSizes=1
  Sum : Sum  Inputs=|+-
  Sum1 : Sum  Inputs=|++
  Sum2 : Sum  Inputs=|+-
  Sum3 : Sum  Inputs=|++
  Sum4 : Sum  Inputs=|++
  Sum5 : Sum  Inputs=++|
  Sum6 : Sum  Inputs=-+|
  Sum7 : Sum  Inputs=++|
  Switch1 : Switch  Criteria=u2 > Threshold
  Switch2 : Switch  Criteria=u2 > Threshold
  i_s_ref_dq0 : Outport  VectorParamsAs1DForOutWhenUnconnected=off
  wires:
  Integration Time3/1 -> Sum4/2
  Integration Time2/1 -> Sum1/2
  Sum/1 -> Integration Time2/1, Integration Time/1
  Mux/1 -> i_s_ref_dq0/1
  Selector2/1 -> Demux2/1
  Selector1/1 -> Demux/1
  Selector/1 -> Demux1/1
  Damping (q)/1 -> Sum5/2  "Is_q\""
  v_dq0/1 -> Selector/1
  Sum3/1 -> Mux/1  "Is_d*"
  Sum4/1 -> Damping (q)/1
  Integrator/1 -> Sum1/1
  Sum1/1 -> Damping (d)/1
  Sum5/1 -> Sum7/2  "Is_q'"
  i_dq0/1 -> Selector2/1
  Damping (d)/1 -> Sum2/1  "Is_d\""
  Filter capacitance/1 -> Eg_d * (wCf)/2, "Eg_q * (wCf) "/2
  Demux1/2 -> Sum6/1, "Eg_q * (wCf) "/1  "Eg_q"
  "Eg_q * (wCf) "/1 -> Sum2/2  "Is_f"
  Current Compensator1/1 -> Sum7/1
  Demux1/1 -> Sum/2, Eg_d * (wCf)/1  "Eg_d"
  Current Compensator/1 -> Sum3/2
  Sum2/1 -> Sum3/1  "Is_d'"
  Demux2/1 -> Current Compensator/1  "Ig_d"
  Sum6/1 -> Integration Time3/1, Integration Time1/1
  Demux/1 -> Sum/1  "Eg_d*"
  Demux2/2 -> Current Compensator1/1  "Ig_q"
  Sum7/1 -> Mux/2  "Is_q*"
  Eg_d * (wCf)/1 -> Sum5/1  "Is_f"
  v_ref_dq0/1 -> Selector1/1
  Demux/2 -> Sum6/2  "Eg_q*"
  Integrator1/1 -> Sum4/1
  w/1 -> Filter capacitance/1
  Is_0*/1 -> Mux/3
  Switch2/1 -> Integrator/1
  Integration Time/1 -> Switch2/1
  anti-windup/1 -> Switch1/2, Switch2/2
  Constant/1 -> Switch2/3
  Switch1/1 -> Integrator1/1
  Constant1/1 -> Switch1/3
  Integration Time1/1 -> Switch1/1

== system ANS_GFM_long_term/OLTC/ OLTC Control ==
  note: The 2 resistors are in operation during TransferTime/3
  note: Tap changer Mechanical Delay= TapSelectionTime
  Up : Inport
  Down : Inport  Port=2
  Abs1 : Abs  SaturateOnIntegerOverflow=on
  Constant : Constant  Value=TapVector
  Edge Detector : spsEdgeDetectorLib/Edge Detector  model=Rising  ic=0  Ts=0
      settings: SourceProductBaseCode=PS
  Logical Operator : Logic  Operator=NOT  AllPortsSameDT=off
  Monostable1 : spsMonostableLib/Monostable  EdgeDetect=Rising  PulseDuration=TransferTime  ic=1  Ts=0
      settings: SourceProductBaseCode=PS
  Off Delay : spsOnDelayLib/On Delay  DelayType=Off delay  delay=2*TransferTime/3  ic=InitialStates  Ts=0
      settings: SourceProductBaseCode=PS
  On Delay : spsOnDelayLib/On Delay  DelayType=On delay  delay=TransferTime/3  ic=1  Ts=0
      settings: SourceProductBaseCode=PS
  Relational Operator : RelationalOperator  Operator===  RndMeth=Nearest
  S-R Flip-Flop : simulink_extras/Flip Flops/S-R Flip-Flop  initial_condition=InitialTap>=0
  Set Reset : Subsystem
  Tap Changer Control : Subsystem  mask(Tap Changer Control){MinMaxTap=[-NumberOfTaps  +NumberOfTaps], InitialPosition=InitialTap, MecDelay=TapSelectionTime}
      mask prompts: MinMaxTap "Minimum and maximum tap number [ Min  Max ] :"; InitialPosition "Initial tap position"; MecDelay "Mechanical delay time"
      mask init:
      | if MecDelay<=0,
      | 	MecDelay=1/60;
      | end
  Terminator1 : Terminator
  Tap : Outport  VectorParamsAs1DForOutWhenUnconnected=off
  SwSelect : Outport  Port=2  VectorParamsAs1DForOutWhenUnconnected=off
  SwTr : Outport  Port=3  VectorParamsAs1DForOutWhenUnconnected=off
  SwInv : Outport  Port=4  VectorParamsAs1DForOutWhenUnconnected=off
  Ready : Outport  Port=5  VectorParamsAs1DForOutWhenUnconnected=off
  wires:
  Constant/1 -> Relational Operator/2
  Logical Operator/1 -> SwTr/1
  Down/1 -> Tap Changer Control/2(Down)
  Up/1 -> Tap Changer Control/1(Up)
  Relational Operator/1 -> On Delay/1
  Monostable1/1 -> Logical Operator/1
  Tap Changer Control/1(TapNo) -> Tap/1, Edge Detector/1, Set Reset/1(Tap), Abs1/1
  Tap Changer Control/2(Ready) -> Ready/1
  S-R Flip-Flop/2 -> Terminator1/1
  Edge Detector/1 -> Monostable1/1
  S-R Flip-Flop/1 -> SwInv/1
  Abs1/1 -> Relational Operator/1
  On Delay/1 -> Off Delay/1
  Off Delay/1 -> SwSelect/1
  Set Reset/1(Set) -> S-R Flip-Flop/1
  Set Reset/2(Reset) -> S-R Flip-Flop/2
